simulink model "torqueMode"  (R2022a)
settings: Solver=FixedStepAuto  StartTime=0.0  StopTime=simTime  FixedStep=sampleTime  RelTol=1e-3
values from neighbouring files (symbols this model uses):
  coulombTorqueNegative = theta(4)/theta(2)    [LeastSquare.m]    (also in leastSquare.m; velRide.m = resultFitNeg(2); velocityRide.m = resultFitNeg(2))
  coulombTorquePositive = theta(3)/theta(2)    [LeastSquare.m]    (also in leastSquare.m; velRide.m = resultFitPos(2); velocityRide.m = resultFitPos(2))
  inertia = 1/K_w    [LeastSquare.m]    (also in leastSquare.m)
  viscousDamping = -inertia*p_w    [LeastSquare.m]    (also in leastSquare.m; velRide.m = (viscousDampingPos+viscousDampingNeg)/2; velocityRide.m = (viscousDampingPos+viscousDampingNeg)/2)
settings Model: Creator=kose  LastModifiedBy=kose
settings DataIOCC: SaveFormat=Array

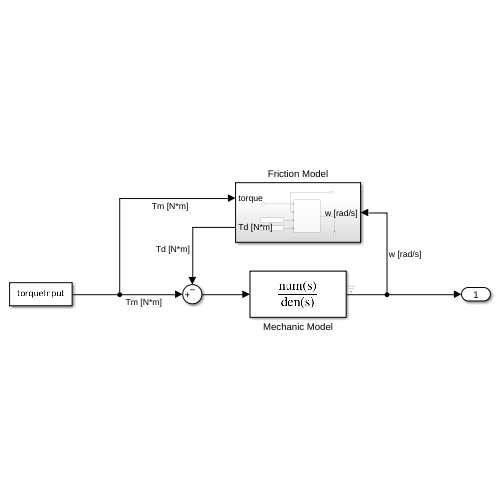
[thumbnail: Simulink's stored preview of the top-level diagram]
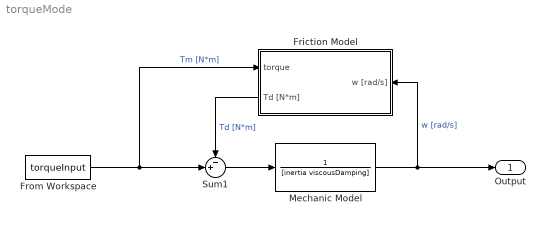
== system torqueMode ==
  Friction Model : Subsystem
      settings: PortSchema="{\"entries\":[{\"content\":{\"sides\":[{\"content\":{\"connectorIds\":[\"In1\"]},\"type\":\"ConnectorPlacement.EquallySpacedRectSide\",\"uuid\":\"8173ecdf-76e4-4809-8dcd-ec0655641a82\"},{\"content\":{\"connectorIds\":[\"In2\",\"Out1\"],\"side\":\"RIGHT\"},\"type\":\"ConnectorPlacement.EquallySpacedRectSide\",\"uuid\":\"02bfb555-c54c-45db-8ee8-f3cb4a7ead24\"},{\"content\":{\"connectorIds\":[],\"side\":\"TOP\"},\"type\":\"ConnectorPlacement.EquallySpacedRectSide\",\"uuid\":\"776da3c7-b053-4a98-8e1b-c60377d5559b\"}]},\"type\":\"ConnectorPlacement.EquallySpacedConnector\",\"uuid\":\"773d656e-d403-490b-8d7a-ce1c081af26d\"}],\"packageUris\":[\"http://schema.mathworks.com/mf0/Connector/R2020b\"],\"version\":\"1.0\"}"
  From Workspace : FromWorkspace  VariableName=torqueInput
  Mechanic Model : TransferFcn  Denominator=[inertia viscousDamping]
  Sum1 : Sum  Inputs=-+|
  Output : Outport
  wires:
  Mechanic Model/1 -> Friction Model/1(w [rad/s]), Output/1  "w [rad/s]"
  From Workspace/1 -> Friction Model/2(torque), Sum1/2  "Tm [N*m]"
  Sum1/1 -> Mechanic Model/1
  Friction Model/1(Td [N*m]) -> Sum1/1  "Td [N*m]"

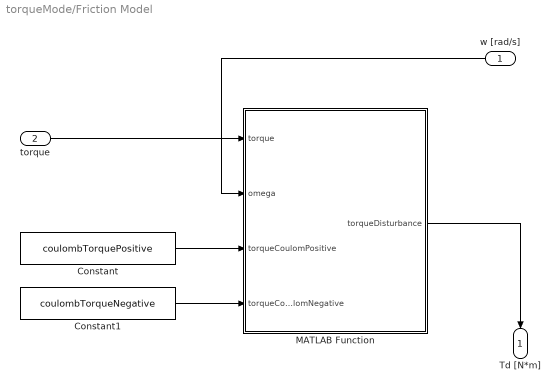
== system torqueMode/Friction Model ==
  w [rad/s] : Inport
  torque : Inport  Port=2
  Constant : Constant  Value=coulombTorquePositive
  Constant1 : Constant  Value=coulombTorqueNegative
  MATLAB Function : MATLAB Function  TreatAsAtomicUnit=on
  Td [N*m] : Outport
  wires:
  w [rad/s]/1 -> MATLAB Function/2(omega)
  Constant/1 -> MATLAB Function/3(torqueCoulomPositive)
  torque/1 -> MATLAB Function/1(torque)
  MATLAB Function/1(torqueDisturbance) -> Td [N*m]/1
  Constant1/1 -> MATLAB Function/4(torqueCoulomNegative)

== matlab function torqueMode/Friction Model/MATLAB Function ==
  data: torque input; torqueDisturbance output; omega input; torqueCoulomPositive input; torqueCoulomNegative input
function torqueDisturbance = fcn(torque, omega, torqueCoulomPositive, torqueCoulomNegative)

if omega > 0
    torqueDisturbance = torqueCoulomPositive;
elseif omega < 0
    torqueDisturbance = torqueCoulomNegative;    
elseif omega == 0 &&  torque < torqueCoulomPositive
    torqueDisturbance = torque;
elseif omega == 0 && torque < torqueCoulomNegative
    torqueDisturbance = torque;
else
    torqueDisturbance = 0;
end
end
